simulink model "PPF_shin"  (R2020b)
settings: Solver=VariableStepAuto  StartTime=0.0  StopTime=10  RelTol=1e-3
settings Model: Creator=xinxinzhang  LastModifiedBy=xinxinzhang

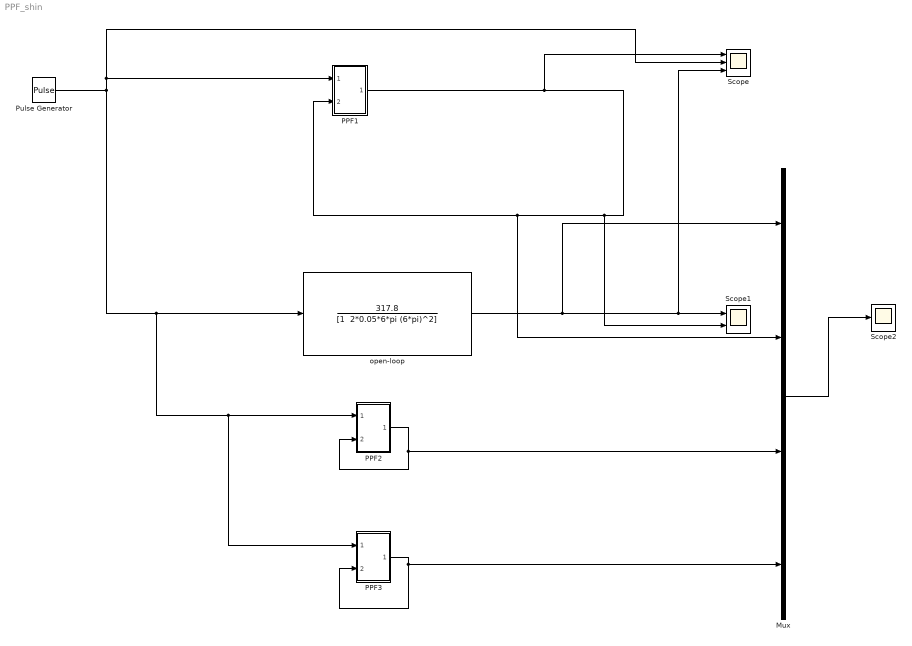
== system PPF_shin ==
  Mux : Mux
  PPF1 : Subsystem
  PPF2 : Subsystem
  PPF3 : Subsystem
  Pulse Generator : DiscretePulseGenerator  PulseType=Time based  Period=20  PulseWidth=0.1
  Scope : Scope  NumInputPorts=3
  Scope1 : Scope  NumInputPorts=2
  Scope2 : Scope
  open-loop : TransferFcn  Numerator=[317.8]  Denominator="[1  2*0.05*6*pi (6*pi)^2]"
  wires:
  Pulse Generator/1 -> PPF1/1(In1), Scope/2, PPF3/1(In1), PPF2/1(In1), open-loop/1
  open-loop/1 -> Mux/1, Scope/3, Scope1/1
  PPF1/1(Out1) -> Scope/1, PPF1/2(In2), Mux/2, Scope1/2
  PPF2/1(Out1) -> PPF2/2(In2), Mux/3
  Mux/1 -> Scope2/1
  PPF3/1(Out1) -> Mux/4, PPF3/2(In2)

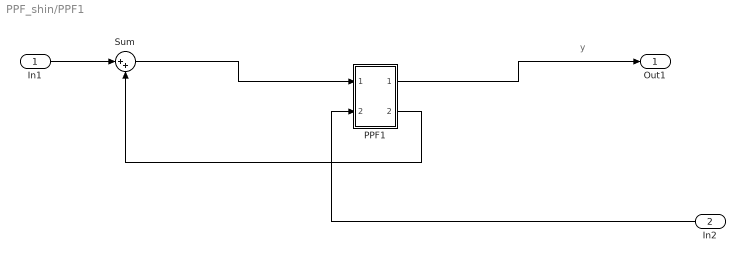
== system PPF_shin/PPF1 ==
  note: y
  In1 : Inport
  In2 : Inport  Port=2
  PPF1 : Subsystem
  Sum : Sum  Inputs=|++
  Out1 : Outport
  wires:
  Sum/1 -> PPF1/1(In1)
  In1/1 -> Sum/1
  PPF1/2(Out2) -> Sum/2
  In2/1 -> PPF1/2(In2)
  PPF1/1(Out1) -> Out1/1

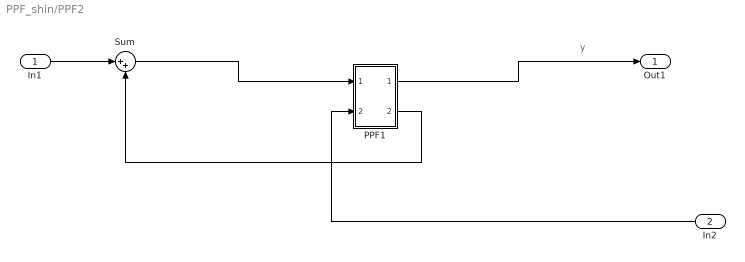
== system PPF_shin/PPF2 ==
  note: y
  In1 : Inport
  In2 : Inport  Port=2
  PPF1 : Subsystem
  Sum : Sum  Inputs=|++
  Out1 : Outport
  wires:
  PPF1/1(Out1) -> Out1/1
  In2/1 -> PPF1/2(In2)
  PPF1/2(Out2) -> Sum/2
  In1/1 -> Sum/1
  Sum/1 -> PPF1/1(In1)

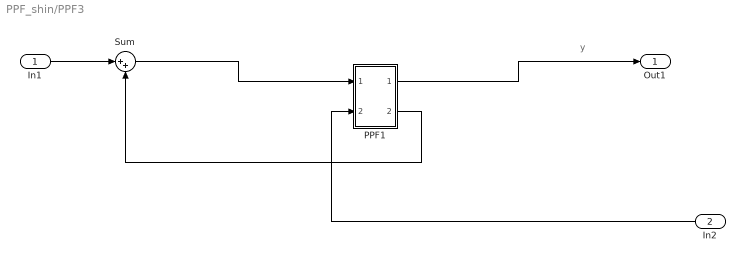
== system PPF_shin/PPF3 ==
  note: y
  In1 : Inport
  In2 : Inport  Port=2
  PPF1 : Subsystem
  Sum : Sum  Inputs=|++
  Out1 : Outport
  wires:
  Sum/1 -> PPF1/1(In1)
  In1/1 -> Sum/1
  PPF1/2(Out2) -> Sum/2
  In2/1 -> PPF1/2(In2)
  PPF1/1(Out1) -> Out1/1

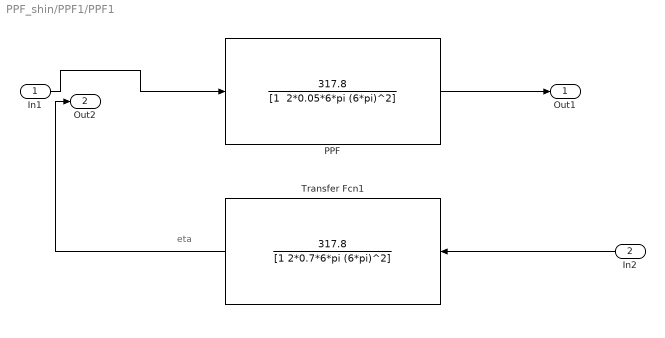
== system PPF_shin/PPF1/PPF1 ==
  note: eta
  In1 : Inport
  In2 : Inport  Port=2
  PPF : TransferFcn  Numerator=[317.8]  Denominator="[1  2*0.05*6*pi (6*pi)^2]"
  Transfer Fcn1 : TransferFcn  Numerator=[317.8]  Denominator=[1 2*0.7*6*pi (6*pi)^2]
  Out1 : Outport
  Out2 : Outport  Port=2
  wires:
  In1/1 -> PPF/1
  PPF/1 -> Out1/1
  In2/1 -> Transfer Fcn1/1
  Transfer Fcn1/1 -> Out2/1

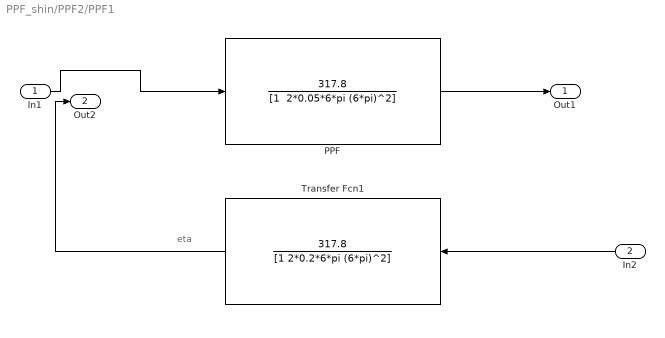
== system PPF_shin/PPF2/PPF1 ==
  note: eta
  In1 : Inport
  In2 : Inport  Port=2
  PPF : TransferFcn  Numerator=[317.8]  Denominator="[1  2*0.05*6*pi (6*pi)^2]"
  Transfer Fcn1 : TransferFcn  Numerator=[317.8]  Denominator=[1 2*0.2*6*pi (6*pi)^2]
  Out1 : Outport
  Out2 : Outport  Port=2
  wires:
  Transfer Fcn1/1 -> Out2/1
  In2/1 -> Transfer Fcn1/1
  PPF/1 -> Out1/1
  In1/1 -> PPF/1

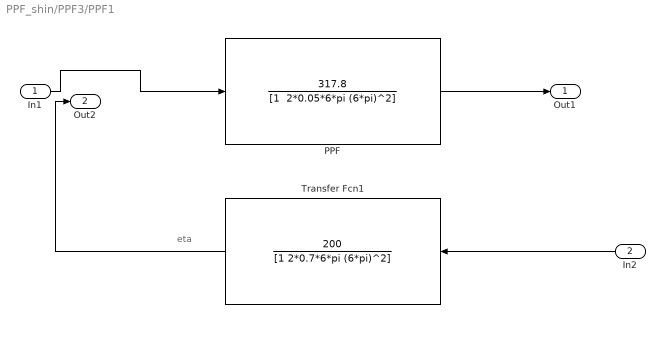
== system PPF_shin/PPF3/PPF1 ==
  note: eta
  In1 : Inport
  In2 : Inport  Port=2
  PPF : TransferFcn  Numerator=[317.8]  Denominator="[1  2*0.05*6*pi (6*pi)^2]"
  Transfer Fcn1 : TransferFcn  Numerator=[200]  Denominator=[1 2*0.7*6*pi (6*pi)^2]
  Out1 : Outport
  Out2 : Outport  Port=2
  wires:
  In1/1 -> PPF/1
  PPF/1 -> Out1/1
  In2/1 -> Transfer Fcn1/1
  Transfer Fcn1/1 -> Out2/1
